simulink model "fan_park"  (R2024b)
settings: Solver=VariableStepAuto  StartTime=0.0  StopTime=10.0  RelTol=1e-3
settings Model: Creator=罗芳成  LastModifiedBy=罗芳成

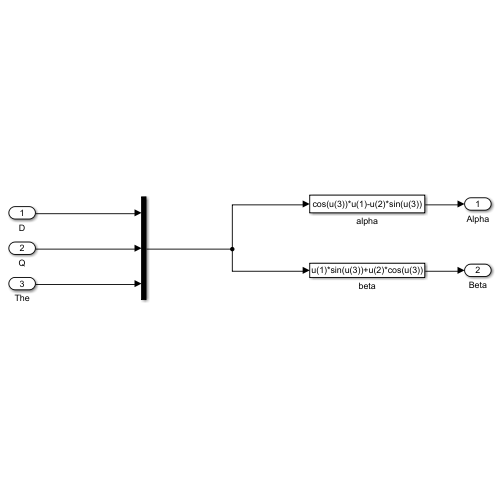
[thumbnail: Simulink's stored preview of the top-level diagram]
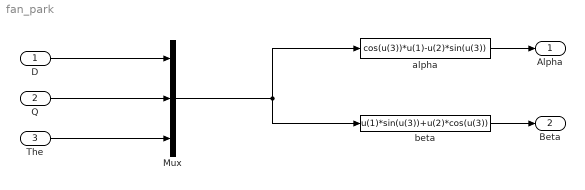
== system fan_park ==
  D : Inport
  Q : Inport  Port=2
  The : Inport  Port=3
  Mux : Mux  Inputs=3
  alpha : Fcn  Expr=cos(u(3))*u(1)-u(2)*sin(u(3))
  beta : Fcn  Expr=u(1)*sin(u(3))+u(2)*cos(u(3))
  Alpha : Outport
  Beta : Outport  Port=2
  wires:
  D/1 -> Mux/1
  Q/1 -> Mux/2
  The/1 -> Mux/3
  Mux/1 -> beta/1, alpha/1
  alpha/1 -> Alpha/1
  beta/1 -> Beta/1
